simulink model "KalmanFilterUnitTestModel"  (R2019b)
settings: Solver=FixedStepDiscrete  StartTime=time_start  StopTime=time_end  FixedStep=dt  RelTol=1e-3
values from neighbouring files (symbols this model uses):
  Q = 0.05    [KalmanFilterUnitTest_dataset.mat]
  R = [0.64  0; 0  0.64]    [KalmanFilterUnitTest_dataset.mat]    (also in compute_variance_covariance_matrix.m = V)
libraries: posefilter x1

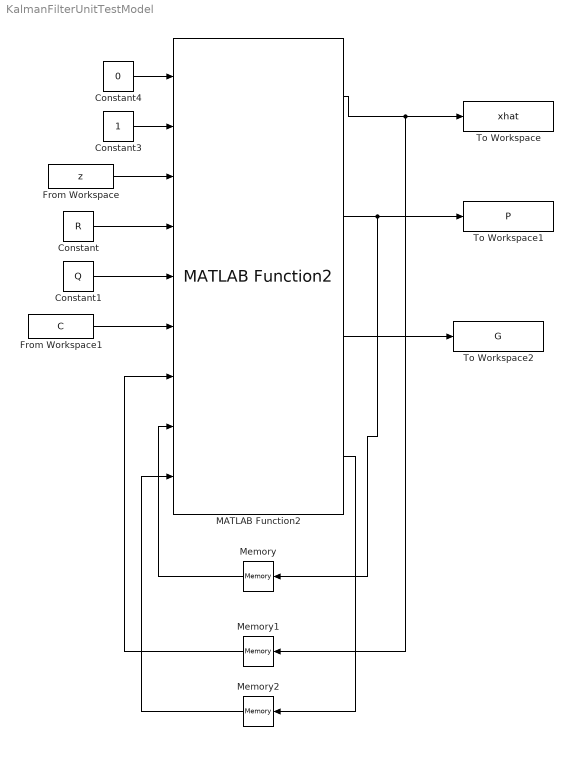
== system KalmanFilterUnitTestModel ==
  Constant : Constant  Value=R
  Constant1 : Constant  Value=Q
  Constant3 : Constant
  Constant4 : Constant  Value=0
  From Workspace : FromWorkspace  VariableName=z  SampleTime=0  Interpolate=off  OutputAfterFinalValue=Setting to zero
  From Workspace1 : FromWorkspace  VariableName=C  SampleTime=0  Interpolate=off  OutputAfterFinalValue=Setting to zero
  MATLAB Function2 : posefilter/MATLAB Function2  SystemSampleTime=-1  Latency=0  AutoFrameSizeCalculation=off
  Memory : Memory  InheritSampleTime=on
  Memory1 : Memory  InheritSampleTime=on
  Memory2 : Memory  InheritSampleTime=on
  To Workspace : ToWorkspace  VariableName=xhat  SaveFormat=Timeseries  SampleTime=-1
  To Workspace1 : ToWorkspace  VariableName=P  SaveFormat=Timeseries  SampleTime=-1
  To Workspace2 : ToWorkspace  VariableName=G  SaveFormat=Timeseries  SampleTime=-1
  wires:
  MATLAB Function2/2 -> To Workspace1/1, Memory/1
  Memory/1 -> MATLAB Function2/8
  MATLAB Function2/1 -> Memory1/1, To Workspace/1
  Memory1/1 -> MATLAB Function2/7
  From Workspace/1 -> MATLAB Function2/3
  Constant/1 -> MATLAB Function2/4
  Constant1/1 -> MATLAB Function2/5
  From Workspace1/1 -> MATLAB Function2/6
  MATLAB Function2/4 -> Memory2/1
  Memory2/1 -> MATLAB Function2/9
  MATLAB Function2/3 -> To Workspace2/1
  Constant3/1 -> MATLAB Function2/2
  Constant4/1 -> MATLAB Function2/1
